simulink model "RI_DIHJ"  (R2013b)
settings: Solver=ode45  StartTime=0.0  StopTime=10.0  RelTol=1e-3
settings Model: Creator=Szalay  LastModifiedBy=Szalay

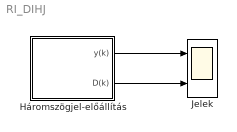
== system RI_DIHJ ==
  Háromszögjel-előállítás : Subsystem  mask{T_S=0.1, N=10}
      mask prompts: T_S "Mintavételi idő"; N "Csúcsérték"
  Jelek : Scope  NumInputPorts=2
      settings: ShowLegends=on  YMin=-5~-5  YMax=5~5
  wires:
  Háromszögjel-előállítás/1(y(k)) -> Jelek/1
  Háromszögjel-előállítás/2(D(k)) -> Jelek/2

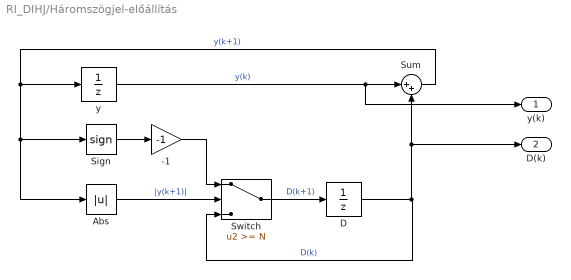
== system RI_DIHJ/Háromszögjel-előállítás ==
  -1 : Gain  Gain=-1
  Abs : Abs
  D : UnitDelay  InitialCondition=-1  SampleTime=T_S
  Sign : Signum
  Sum : Sum  Inputs=|++
  Switch : Switch  Threshold=N
  y : UnitDelay  InitialCondition=N  SampleTime=T_S
  y(k) : Outport
  D(k) : Outport  Port=2
  wires:
  Abs/1 -> Switch/2  "|y(k+1)|"
  D/1 -> Sum/2, D(k)/1, Switch/3  "D(k)"
  Sign/1 -> -1/1
  y/1 -> y(k)/1, Sum/1  "y(k)"
  Switch/1 -> D/1  "D(k+1)"
  Sum/1 -> y/1, Sign/1, Abs/1  "y(k+1)"
  -1/1 -> Switch/1
